simulink model "dpsk"  (R2017a)
settings: Solver=VariableStepAuto  StartTime=0.0  StopTime=10  RelTol=1e-3
libraries: commdigbbndpm3 x2, commchan3 x1, commrandsrc3 x1
settings Model: Creator=Vibha  LastModifiedBy=Vibha

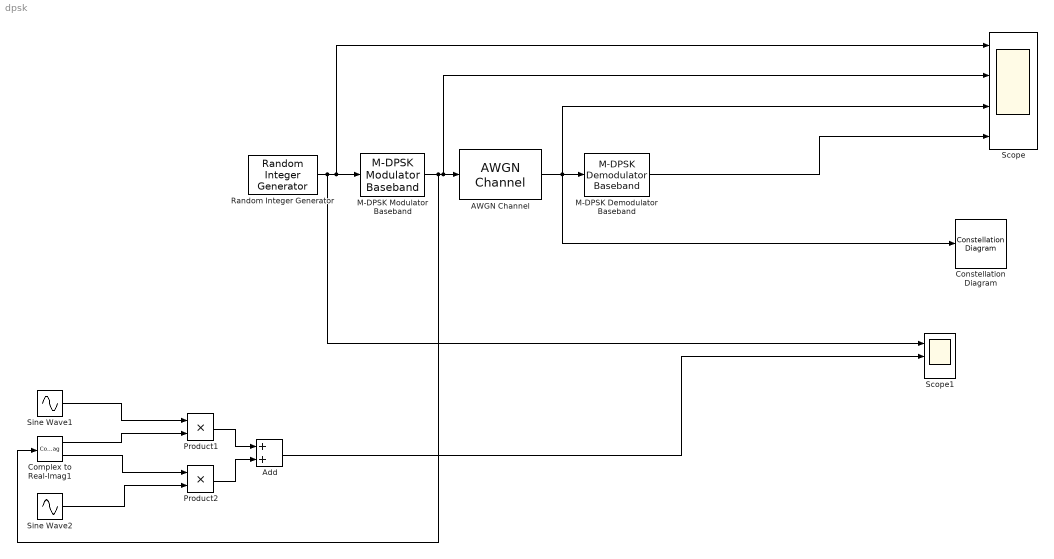
== system dpsk ==
  AWGN Channel : commchan3/AWGN Channel  InputProcessing=Columns as channels (frame based)  seed=67  noiseMode="Signal to noise ratio  (Eb/No)"  EbNodB=10  EsNodB=10  SNRdB=10  bitsPerSym=2  Ps=1  Tsym=1  variance=1
  Add : Sum
  Complex to Real-Imag1 : ComplexToRealImag
  Constellation Diagram : ConstellationDiagram
  M-DPSK Demodulator Baseband : commdigbbndpm3/M-DPSK Demodulator Baseband  M=2  OutType=Integer  Dec=Gray  Ph=pi  outDtype1=Inherit via internal rule  outDtype2=Inherit via internal rule
      settings: SourceProductName=Communications System Toolbox  SourceProductBaseCode=CM
  M-DPSK Modulator Baseband : commdigbbndpm3/M-DPSK Modulator Baseband  M=2  InType=Integer  Enc=Binary  Ph=pi  outDtype=double
      settings: SourceProductName=Communications System Toolbox  SourceProductBaseCode=CM
  Product1 : Product
  Product2 : Product
  Random Integer Generator : commrandsrc3/Random Integer Generator  SetSize=2  SeedSource=Parameter  Seed=37  SampleTime=1  SamplesPerFrame=1  OutputDataType=double  SimulateUsing=Interpreted execution
  Scope : Scope  NumInputPorts=4
  Scope1 : Scope  NumInputPorts=3
  Sine Wave1 : Sin  Amplitude=4  Frequency=4*2*pi  SampleTime=0.001  VectorParams1D=off
  Sine Wave2 : Sin  Amplitude=4  Frequency=4*2*pi  Phase=pi/2  SampleTime=0.001  VectorParams1D=off
  wires:
  AWGN Channel/1 -> M-DPSK Demodulator Baseband/1, Constellation Diagram/1, Scope/3
  M-DPSK Demodulator Baseband/1 -> Scope/4
  M-DPSK Modulator Baseband/1 -> Complex to Real-Imag1/1, Scope/2, AWGN Channel/1
  Product1/1 -> Add/1
  Product2/1 -> Add/2
  Complex to Real-Imag1/2 -> Product2/1
  Complex to Real-Imag1/1 -> Product1/2
  Random Integer Generator/1 -> Scope1/1, Scope/1, M-DPSK Modulator Baseband/1
  Sine Wave1/1 -> Product1/1
  Sine Wave2/1 -> Product2/2
  Add/1 -> Scope1/2
